simulink model "Non_linear_model"  (R2019b)
settings: Solver=VariableStepAuto  StartTime=0.0  StopTime=15  RelTol=1e-6
undefined symbols (not defined in the file or in its folder): D0, E0, I0, J0, R0, S0, u_val
settings Model: Creator=felipeareces  LastModifiedBy=felipeareces

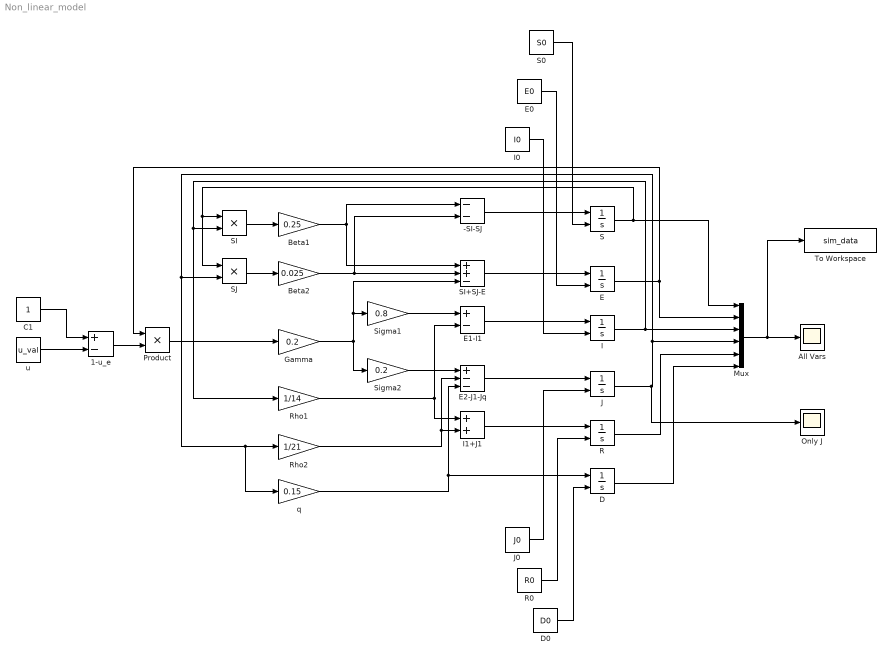
== system Non_linear_model ==
  -SI-SJ : Sum  Inputs=--
  1-u_e : Sum  Inputs=+-
  All Vars : Scope
  Beta1 : Gain  Gain=0.25
  Beta2 : Gain  Gain=0.025
  C1 : Constant
  D : Integrator  InitialConditionSource=external
  D0 : Constant  Value=D0
  E : Integrator  InitialConditionSource=external
  E0 : Constant  Value=E0
  E1-I1 : Sum  Inputs=+-
  E2-J1-Jq : Sum  Inputs=+--
  Gamma : Gain  Gain=0.2
  I : Integrator  InitialConditionSource=external
  I0 : Constant  Value=I0
  I1+J1 : Sum
  J : Integrator  InitialConditionSource=external
  J0 : Constant  Value=J0
  Mux : Mux  Inputs=6
  Only J : Scope
  Product : Product
  R : Integrator  InitialConditionSource=external
  R0 : Constant  Value=R0
  Rho1 : Gain  Gain=1/14
  Rho2 : Gain  Gain=1/21
  S : Integrator  InitialConditionSource=external
  S0 : Constant  Value=S0
  SI : Product
  SI+SJ-E : Sum  Inputs=++-
  SJ : Product
  Sigma1 : Gain  Gain=0.8
  Sigma2 : Gain  Gain=0.2
  To Workspace : ToWorkspace  VariableName=sim_data  SaveFormat=Timeseries  SampleTime=-1
  q : Gain  Gain=0.15
  u : Constant  Value=u_val
  wires:
  S0/1 -> S/2
  E0/1 -> E/2
  D0/1 -> D/2
  R0/1 -> R/2
  J0/1 -> J/2
  I0/1 -> I/2
  S/1 -> Mux/1, SJ/1, SI/1
  I/1 -> Mux/3, Rho1/1, SI/2
  SI/1 -> Beta1/1
  J/1 -> Only J/1, Mux/4, q/1, Rho2/1, SJ/2
  SJ/1 -> Beta2/1
  -SI-SJ/1 -> S/1
  Beta1/1 -> SI+SJ-E/1, -SI-SJ/1
  Beta2/1 -> -SI-SJ/2, SI+SJ-E/2
  Gamma/1 -> Sigma2/1, SI+SJ-E/3, Sigma1/1
  E/1 -> Product/1, Mux/2
  SI+SJ-E/1 -> E/1
  Sigma1/1 -> E1-I1/1
  E1-I1/1 -> I/1
  Rho1/1 -> E1-I1/2, I1+J1/1
  Sigma2/1 -> E2-J1-Jq/1
  Rho2/1 -> E2-J1-Jq/2, I1+J1/2
  q/1 -> E2-J1-Jq/3, D/1
  R/1 -> Mux/5
  D/1 -> Mux/6
  I1+J1/1 -> R/1
  E2-J1-Jq/1 -> J/1
  Mux/1 -> To Workspace/1, All Vars/1
  u/1 -> 1-u_e/2
  C1/1 -> 1-u_e/1
  1-u_e/1 -> Product/2
  Product/1 -> Gamma/1
